simulink model "func3_a"  (R2016a)
settings: Solver=VariableStepAuto  StartTime=0.0  StopTime=10.0  RelTol=1e-3
libraries: ModelComposer x2, basics_3_lib x1
settings Model: Creator=abehbood  LastModifiedBy=abehbood
settings GRTTargetCC: GeneratePreprocessorConditionals=Use local settings

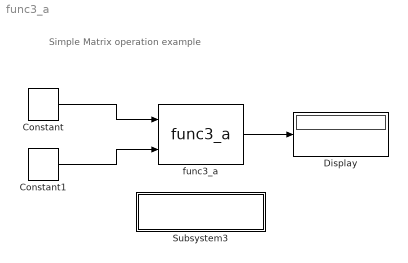
== system func3_a ==
  note: Simple Matrix operation example
  Constant : ModelComposer/Constant  Value=[1,2,3,2,1;1,4,1,1,4;1,2,1,2,1]  SampleTime=1.0  OutDataType=int16  TypeExp=''  Signedness=Signed  WordLength=16  FractionalLength=0  RoundingMode=Truncation to minus infinity  OverflowMode=Wrap around
  Constant1 : ModelComposer/Constant  Value=[1,2,3,2,1;1,4,1,1,4;1,2,1,2,1]  SampleTime=1.0  OutDataType=int16  TypeExp=''  Signedness=Signed  WordLength=16  FractionalLength=0  RoundingMode=Truncation to minus infinity  OverflowMode=Wrap around
  Display : Display
  Subsystem3 : Subsystem
      settings: OpenFcn=xmcOpenFileEx
      mask Display: disp(sprintf('Double Click to open\nthe main header file'))
  func3_a : basics_3_lib/func3_a  LibraryFunction=func3_a  IncludeFiles={'func3_a.h'}  SourceFiles={}  IncludeDirectories={}  TemplateParams={' '}  FunctionParamTypes={xmcDataType('void'); xmcDataType('const int16_t'); xmcDataType('const int16_t'); xmcDataType('int16_t')}  FunctionParamPassbys={0.000000000000000000e+00; 0.000000000000000000e+00; 0.000000000000000000e+00; 0.000000000000000000e+00}  FunctionParamDimensions={'1'; '[3][5]'; '[3][5]'; '[3][5]'}  FunctionParamNames={'return'; 'in1'; 'in2'; 'out'}  FunctionParamDir={0.000000000000000000e+00; 1.000000000000000000e+00; 1.000000000000000000e+00; 2.000000000000000000e+00}  FunctionParamSupportsStreaming={false; false; false; false}  BufferDepth={'0'}  FunctionParamValues={'0'; '0'; '0'; '0'}
  wires:
  Constant/1 -> func3_a/1
  func3_a/1 -> Display/1
  Constant1/1 -> func3_a/2

== system func3_a/Subsystem3 ==
